simulink model "scara_brush"  (R2026a)
settings: Solver=ode4  StopTime=scara_ref.t(end)  FixedStep=scara_p.dt
InitFcn:
  | addpath(fileparts(fileparts(fileparts(get_param(bdroot,'FileName'))))); startup_scara(); scara_setup();
undefined symbols (not defined in the file): scara_q0
settings Model: Creator=vutua  LastModifiedBy=vutua

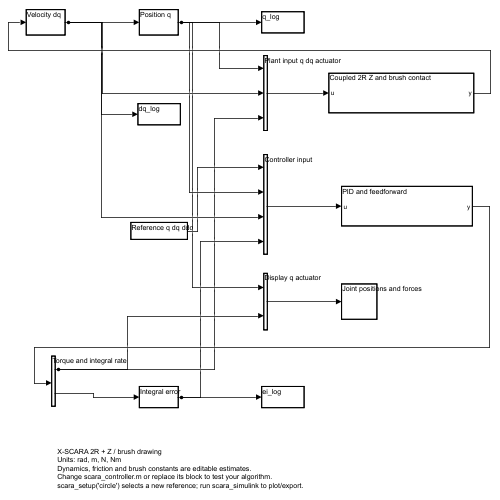
[thumbnail: Simulink's stored preview of the top-level diagram]
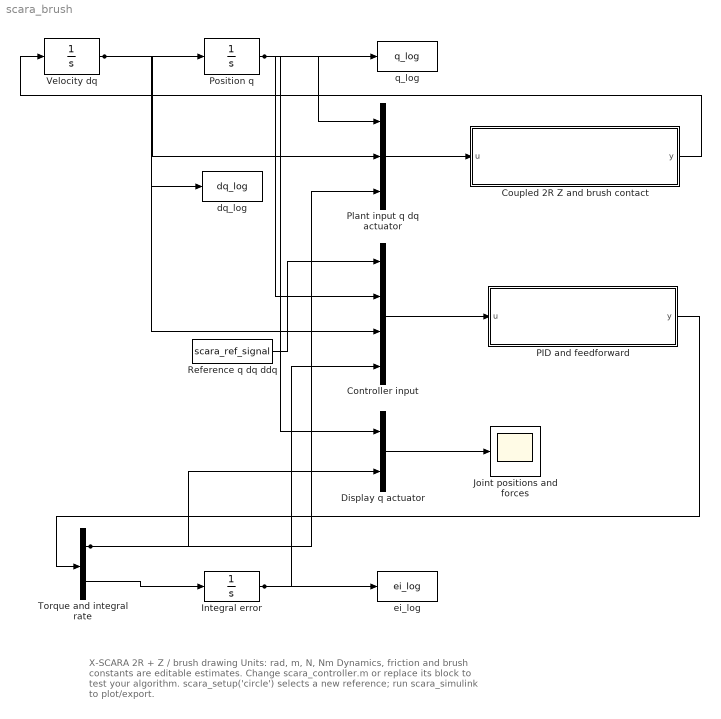
== system scara_brush ==
  note: X-SCARA 2R + Z / brush drawing
      | Units: rad, m, N, Nm
      | Dynamics, friction and brush constants are editable estimates.
      | Change scara_controller.m or replace its block to test your algorithm.
      | scara_setup('circle') selects a new reference; run scara_simulink to plot/export.
  Controller input : Mux
  Coupled 2R Z and brush contact : MATLAB Function  TreatAsAtomicUnit=on
  Display q actuator : Mux  Inputs=2
  Integral error : Integrator  InitialCondition=[0;0;0]
  Joint positions and forces : Scope
  PID and feedforward : MATLAB Function  TreatAsAtomicUnit=on
  Plant input q dq actuator : Mux  Inputs=3
  Position q : Integrator  InitialCondition=scara_q0
  Reference q dq ddq : FromWorkspace  VariableName=scara_ref_signal
  Torque and integral rate : Demux  Outputs=[3 3]
  Velocity dq : Integrator  InitialCondition=[0;0;0]
  dq_log : ToWorkspace  VariableName=dq_log  SampleTime=-1
  ei_log : ToWorkspace  VariableName=ei_log  SampleTime=-1
  q_log : ToWorkspace  VariableName=q_log  SampleTime=-1
  wires:
  Velocity dq/1 -> Plant input q dq actuator/2, Controller input/3, Position q/1, dq_log/1
  Controller input/1 -> PID and feedforward/1(u)
  Torque and integral rate/1 -> Display q actuator/2, Plant input q dq actuator/3
  Reference q dq ddq/1 -> Controller input/1
  Torque and integral rate/2 -> Integral error/1
  Position q/1 -> Controller input/2, Plant input q dq actuator/1, Display q actuator/1, q_log/1
  Integral error/1 -> Controller input/4, ei_log/1
  Plant input q dq actuator/1 -> Coupled 2R Z and brush contact/1(u)
  Display q actuator/1 -> Joint positions and forces/1
  Coupled 2R Z and brush contact/1(y) -> Velocity dq/1
  PID and feedforward/1(y) -> Torque and integral rate/1

== matlab function scara_brush/PID and feedforward ==
  data: u input size=18; y output size=6; scara_numeric_p parameter
function y = fcn(u,scara_numeric_p)
%#codegen
y = scara_controller(u,scara_numeric_p);
end

== matlab function scara_brush/Coupled 2R Z and brush contact ==
  data: u input size=9; y output size=3; scara_numeric_p parameter
function y = fcn(u,scara_numeric_p)
%#codegen
y = scara_accel(u,scara_numeric_p);
end
